simulink library "RIO_Lib"  (R2024b)
settings: Solver=VariableStepAuto  StartTime=0.0  StopTime=10.0  RelTol=1e-3
settings Model: Creator=pepev  LastModifiedBy=pepev

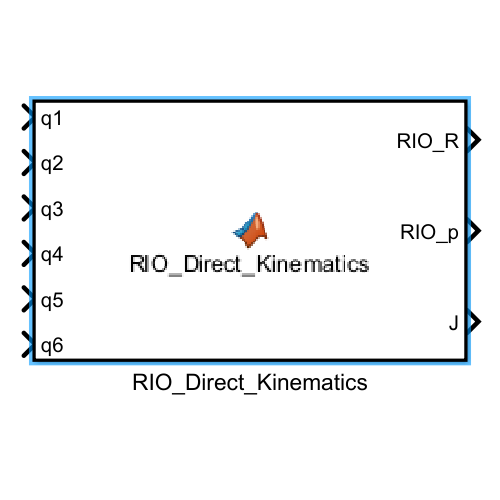
[thumbnail: Simulink's stored preview of the top-level diagram]
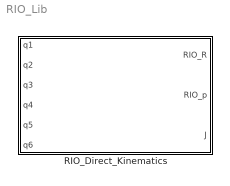
== system RIO_Lib ==
  RIO_Direct_Kinematics : MATLAB Function  TreatAsAtomicUnit=on

== matlab function RIO_Lib/RIO_Direct_Kinematics ==
  data: q1 input; RIO_R output; q2 input; q3 input; q4 input; q5 input; q6 input; RIO_p output; J output
function [RIO_R,RIO_p,J] = RIO_Direct_Kinematics(q1,q2,q3,q4,q5,q6)
%#codegen

%    This function was generated by the Symbolic Math Toolbox version 24.2.
%    20-May-2025 17:05:48

% q1 = complex(q1);  % if required to enforce complex operations
% q2 = complex(q2);  % if required to enforce complex operations
% q3 = complex(q3);  % if required to enforce complex operations
% q4 = complex(q4);  % if required to enforce complex operations
% q5 = complex(q5);  % if required to enforce complex operations
% q6 = complex(q6);  % if required to enforce complex operations
t2 = cos(q1);
t3 = cos(q2);
t4 = cos(q3);
t5 = cos(q4);
t6 = cos(q5);
t7 = cos(q6);
t8 = sin(q1);
t9 = sin(q2);
t10 = sin(q3);
t11 = sin(q4);
t12 = sin(q5);
t13 = sin(q6);
t14 = sqrt(2.0);
t15 = t9.*(3.0./1.0e+1);
t16 = t14+2.0;
t17 = (t9.*t11)./2.0;
t18 = -t14;
t19 = t2.*t3.*(3.0./1.0e+1);
t20 = t3.*t8.*(3.0./1.0e+1);
t21 = (t5.*t9)./1.0e+1;
t24 = (t2.*t4.*t5)./2.0;
t25 = (t2.*t3.*t11)./2.0;
t26 = (t4.*t5.*t8)./2.0;
t27 = (t3.*t5.*t10)./2.0;
t28 = (t3.*t8.*t11)./2.0;
t30 = (t2.*t3.*t5)./1.0e+1;
t31 = (t3.*t4.*t6)./1.0e+1;
t32 = (t3.*t5.*t8)./1.0e+1;
t33 = (t2.*t4.*t11)./1.0e+1;
t34 = (t2.*t6.*t10)./1.0e+1;
t36 = (t4.*t8.*t11)./1.0e+1;
t37 = (t3.*t10.*t11)./1.0e+1;
t38 = (t6.*t8.*t10)./1.0e+1;
t40 = (t2.*t5.*t9.*t10)./2.0;
t42 = (t5.*t8.*t9.*t10)./2.0;
t46 = (t2.*t4.*t6.*t9)./1.0e+1;
t48 = (t4.*t6.*t8.*t9)./1.0e+1;
t51 = (t2.*t9.*t10.*t11)./1.0e+1;
t54 = (t8.*t9.*t10.*t11)./1.0e+1;
t57 = t3.*t5.*t8.*t12.*(-1.0./1.0e+1);
t58 = t2.*t4.*t11.*t12.*(-1.0./1.0e+1);
t59 = t3.*t10.*t11.*t12.*(-1.0./1.0e+1);
t63 = t8.*t9.*t10.*t11.*t12.*(-1.0./1.0e+1);
t22 = -t20;
t23 = t18+2.0;
t29 = sqrt(t16);
t35 = -t28;
t39 = t12.*t21;
t41 = -t31;
t43 = -t32;
t44 = -t33;
t45 = -t37;
t47 = t12.*t30;
t50 = t12.*t33;
t52 = t12.*t36;
t56 = -t48;
t60 = -t54;
t61 = t12.*t51;
t55 = sqrt(t23);
mt1 = [t2.*t4.*t5.*t7-t3.*t7.*t8.*t11-t2.*t10.*t12.*t13-t3.*t5.*t6.*t8.*t13-t2.*t4.*t6.*t11.*t13+t5.*t7.*t8.*t9.*t10+t4.*t8.*t9.*t12.*t13-t6.*t8.*t9.*t10.*t11.*t13,t2.*t3.*t7.*t11+t4.*t5.*t7.*t8-t8.*t10.*t12.*t13+t2.*t3.*t5.*t6.*t13-t2.*t5.*t7.*t9.*t10-t2.*t4.*t9.*t12.*t13-t4.*t6.*t8.*t11.*t13+t2.*t6.*t9.*t10.*t11.*t13,t7.*t9.*t11+t3.*t5.*t7.*t10+t3.*t4.*t12.*t13+t5.*t6.*t9.*t13-t3.*t6.*t10.*t11.*t13];
mt2 = [t13.*t28.*t55-(t2.*t6.*t10.*t29)./2.0+(t4.*t6.*t8.*t9.*t29)./2.0+(t3.*t5.*t8.*t12.*t29)./2.0+(t2.*t4.*t11.*t12.*t29)./2.0+t8.*t10.*t12.*t17.*t29-(t2.*t4.*t5.*t13.*t55)./2.0-(t2.*t7.*t10.*t12.*t55)./2.0-(t3.*t5.*t6.*t7.*t8.*t55)./2.0-(t2.*t4.*t6.*t7.*t11.*t55)./2.0+(t4.*t7.*t8.*t9.*t12.*t55)./2.0-(t5.*t8.*t9.*t10.*t13.*t55)./2.0-(t6.*t7.*t8.*t9.*t10.*t11.*t55)./2.0];
mt3 = [t13.*t40.*t55-(t6.*t8.*t10.*t29)./2.0-(t2.*t4.*t6.*t9.*t29)./2.0-(t2.*t3.*t5.*t12.*t29)./2.0+(t4.*t8.*t11.*t12.*t29)./2.0-(t2.*t3.*t11.*t13.*t55)./2.0-(t4.*t5.*t8.*t13.*t55)./2.0-(t7.*t8.*t10.*t12.*t55)./2.0-(t2.*t9.*t10.*t11.*t12.*t29)./2.0+(t2.*t3.*t5.*t6.*t7.*t55)./2.0-(t2.*t4.*t7.*t9.*t12.*t55)./2.0-(t4.*t6.*t7.*t8.*t11.*t55)./2.0+t2.*t6.*t7.*t10.*t17.*t55,(t3.*t4.*t6.*t29)./2.0-(t5.*t9.*t12.*t29)./2.0-(t9.*t11.*t13.*t55)./2.0+(t3.*t10.*t11.*t12.*t29)./2.0+(t3.*t4.*t7.*t12.*t55)./2.0+(t5.*t6.*t7.*t9.*t55)./2.0-(t3.*t5.*t10.*t13.*t55)./2.0-(t3.*t6.*t7.*t10.*t11.*t55)./2.0];
mt4 = [t13.*t24.*t29+t13.*t29.*t42-(t2.*t6.*t10.*t55)./2.0+(t2.*t7.*t10.*t12.*t29)./2.0-(t3.*t8.*t11.*t13.*t29)./2.0+(t4.*t6.*t8.*t9.*t55)./2.0+(t3.*t5.*t8.*t12.*t55)./2.0+(t2.*t4.*t11.*t12.*t55)./2.0+t8.*t10.*t12.*t17.*t55+(t3.*t5.*t6.*t7.*t8.*t29)./2.0+(t2.*t4.*t6.*t7.*t11.*t29)./2.0-(t4.*t7.*t8.*t9.*t12.*t29)./2.0+t6.*t7.*t8.*t10.*t17.*t29];
mt5 = [t13.*t25.*t29+t13.*t26.*t29-(t6.*t8.*t10.*t55)./2.0+(t7.*t8.*t10.*t12.*t29)./2.0-(t2.*t4.*t6.*t9.*t55)./2.0-(t2.*t3.*t5.*t12.*t55)./2.0+(t4.*t8.*t11.*t12.*t55)./2.0-(t2.*t3.*t5.*t6.*t7.*t29)./2.0+(t2.*t4.*t7.*t9.*t12.*t29)./2.0+(t4.*t6.*t7.*t8.*t11.*t29)./2.0-(t2.*t5.*t9.*t10.*t13.*t29)./2.0-(t2.*t9.*t10.*t11.*t12.*t55)./2.0-(t2.*t6.*t7.*t9.*t10.*t11.*t29)./2.0,t13.*t17.*t29+t13.*t27.*t29+(t3.*t4.*t6.*t55)./2.0-(t5.*t9.*t12.*t55)./2.0-(t3.*t4.*t7.*t12.*t29)./2.0-(t5.*t6.*t7.*t9.*t29)./2.0+(t3.*t10.*t11.*t12.*t55)./2.0+(t3.*t6.*t7.*t10.*t11.*t29)./2.0];
RIO_R = reshape([mt1,mt2,mt3,mt4,mt5],3,3);
if nargout > 1
    t64 = t9.*t11.*t13.*t29.*(2.3e+1./4.0e+2);
    t65 = t2.*t4.*t5.*t13.*t29.*(2.3e+1./4.0e+2);
    t66 = t3.*t4.*t7.*t12.*t29.*(2.3e+1./4.0e+2);
    t67 = t5.*t6.*t7.*t9.*t29.*(2.3e+1./4.0e+2);
    t68 = t2.*t3.*t11.*t13.*t29.*(2.3e+1./4.0e+2);
    t69 = t4.*t5.*t8.*t13.*t29.*(2.3e+1./4.0e+2);
    t70 = t2.*t7.*t10.*t12.*t29.*(2.3e+1./4.0e+2);
    t71 = t3.*t5.*t10.*t13.*t29.*(2.3e+1./4.0e+2);
    t72 = t3.*t8.*t11.*t13.*t29.*(2.3e+1./4.0e+2);
    t73 = t7.*t8.*t10.*t12.*t29.*(2.3e+1./4.0e+2);
    t83 = t2.*t3.*t5.*t6.*t7.*t29.*(2.3e+1./4.0e+2);
    t84 = t3.*t5.*t6.*t7.*t8.*t29.*(2.3e+1./4.0e+2);
    t85 = t2.*t4.*t6.*t7.*t11.*t29.*(2.3e+1./4.0e+2);
    t86 = t2.*t4.*t7.*t9.*t12.*t29.*(2.3e+1./4.0e+2);
    t87 = t4.*t6.*t7.*t8.*t11.*t29.*(2.3e+1./4.0e+2);
    t88 = t3.*t6.*t7.*t10.*t11.*t29.*(2.3e+1./4.0e+2);
    t89 = t2.*t5.*t9.*t10.*t13.*t29.*(2.3e+1./4.0e+2);
    t90 = t4.*t7.*t8.*t9.*t12.*t29.*(2.3e+1./4.0e+2);
    t91 = t5.*t8.*t9.*t10.*t13.*t29.*(2.3e+1./4.0e+2);
    t100 = t2.*t6.*t7.*t9.*t10.*t11.*t29.*(2.3e+1./4.0e+2);
    t101 = t6.*t7.*t8.*t9.*t10.*t11.*t29.*(2.3e+1./4.0e+2);
    t74 = t3.*t4.*t6.*t55.*(2.3e+1./4.0e+2);
    t75 = t2.*t6.*t10.*t55.*(2.3e+1./4.0e+2);
    t76 = t6.*t8.*t10.*t55.*(2.3e+1./4.0e+2);
    t77 = t5.*t9.*t12.*t55.*(2.3e+1./4.0e+2);
    t78 = -t66;
    t79 = -t67;
    t80 = -t72;
    t92 = t2.*t4.*t6.*t9.*t55.*(2.3e+1./4.0e+2);
    t93 = t2.*t3.*t5.*t12.*t55.*(2.3e+1./4.0e+2);
    t94 = t4.*t6.*t8.*t9.*t55.*(2.3e+1./4.0e+2);
    t95 = t3.*t5.*t8.*t12.*t55.*(2.3e+1./4.0e+2);
    t96 = t2.*t4.*t11.*t12.*t55.*(2.3e+1./4.0e+2);
    t97 = t4.*t8.*t11.*t12.*t55.*(2.3e+1./4.0e+2);
    t98 = t3.*t10.*t11.*t12.*t55.*(2.3e+1./4.0e+2);
    t99 = -t90;
    t102 = t2.*t9.*t10.*t11.*t12.*t55.*(2.3e+1./4.0e+2);
    t103 = t8.*t9.*t10.*t11.*t12.*t55.*(2.3e+1./4.0e+2);
    t81 = -t75;
    t82 = -t77;
    t104 = t15+t17+t21+t27+t39+t41+t45+t59+t64+t71+t74+t78+t79+t82+t88+t98;
    t105 = t22+t24+t34+t35+t42+t43+t44+t56+t57+t58+t60+t63+t65+t70+t80+t81+t84+t85+t91+t94+t95+t96+t99+t101+t103;
    RIO_p = [t105;t19+t25+t26+t30-t36+t38-t40+t46+t47+t51+t61+t68+t69+t73-t76-t83+t86+t87-t89-t92-t93+t97-t100-t102-(t4.*t8.*t11.*t12)./1.0e+1;t104];
end
if nargout > 2
    mt6 = [-t19-t25-t26-t30+t36-t38+t40-t46-t51+t52-t68-t69-t73+t76+t83-t86-t87+t89+t92+t93-t97+t100+t102-(t2.*t3.*t5.*t12)./1.0e+1-(t2.*t9.*t10.*t11.*t12)./1.0e+1,t105,0.0,0.0,0.0,1.0,t8.*t104,-t2.*t104];
    mt7 = [t3.*(3.0./1.0e+1)+(t3.*t5)./1.0e+1+(t3.*t11)./2.0+(t4.*t6.*t9)./1.0e+1+(t3.*t5.*t12)./1.0e+1-(t5.*t9.*t10)./2.0+(t9.*t10.*t11)./1.0e+1+(t9.*t10.*t11.*t12)./1.0e+1+t3.*t11.*t13.*t29.*(2.3e+1./4.0e+2)-t4.*t6.*t9.*t55.*(2.3e+1./4.0e+2)-t3.*t5.*t12.*t55.*(2.3e+1./4.0e+2)-t3.*t5.*t6.*t7.*t29.*(2.3e+1./4.0e+2)+t4.*t7.*t9.*t12.*t29.*(2.3e+1./4.0e+2)-t5.*t9.*t10.*t13.*t29.*(2.3e+1./4.0e+2)-t9.*t10.*t11.*t12.*t55.*(2.3e+1./4.0e+2)-t6.*t7.*t9.*t10.*t11.*t29.*(2.3e+1./4.0e+2),t2,t8,0.0];
    mt8 = [t9.*t26+t9.*t38+t9.*t69+t9.*t73+t9.*t87+t9.*t97+(t2.*t4.*t6)./1.0e+1-(t2.*t5.*t10)./2.0+(t2.*t10.*t11)./1.0e+1-(t4.*t8.*t9.*t11)./1.0e+1+(t2.*t10.*t11.*t12)./1.0e+1-t2.*t4.*t6.*t55.*(2.3e+1./4.0e+2)-(t4.*t8.*t9.*t11.*t12)./1.0e+1+t2.*t4.*t7.*t12.*t29.*(2.3e+1./4.0e+2)-t2.*t5.*t10.*t13.*t29.*(2.3e+1./4.0e+2)-t6.*t8.*t9.*t10.*t55.*(2.3e+1./4.0e+2)-t2.*t10.*t11.*t12.*t55.*(2.3e+1./4.0e+2)-t2.*t6.*t7.*t10.*t11.*t29.*(2.3e+1./4.0e+2)];
    mt9 = [t9.*t33+t9.*t50+t9.*t75+(t4.*t6.*t8)./1.0e+1-(t5.*t8.*t10)./2.0+(t8.*t10.*t11)./1.0e+1-(t2.*t4.*t5.*t9)./2.0-(t2.*t6.*t9.*t10)./1.0e+1+(t8.*t10.*t11.*t12)./1.0e+1-t4.*t6.*t8.*t55.*(2.3e+1./4.0e+2)+t4.*t7.*t8.*t12.*t29.*(2.3e+1./4.0e+2)-t5.*t8.*t10.*t13.*t29.*(2.3e+1./4.0e+2)-t8.*t10.*t11.*t12.*t55.*(2.3e+1./4.0e+2)-t2.*t4.*t5.*t9.*t13.*t29.*(2.3e+1./4.0e+2)-t2.*t7.*t9.*t10.*t12.*t29.*(2.3e+1./4.0e+2)-t6.*t7.*t8.*t10.*t11.*t29.*(2.3e+1./4.0e+2)-t2.*t4.*t9.*t11.*t12.*t55.*(2.3e+1./4.0e+2)-t2.*t4.*t6.*t7.*t9.*t11.*t29.*(2.3e+1./4.0e+2)];
    mt10 = [(t3.*(t4.*t5.*2.0e+2-t4.*t11.*4.0e+1+t6.*t10.*4.0e+1-t4.*t11.*t12.*4.0e+1-t6.*t10.*t55.*2.3e+1+t4.*t5.*t13.*t29.*2.3e+1+t7.*t10.*t12.*t29.*2.3e+1+t4.*t11.*t12.*t55.*2.3e+1+t4.*t6.*t7.*t11.*t29.*2.3e+1))./4.0e+2,t3.*t8,-t2.*t3,-t9];
    mt11 = [t2.*t4.*t5.*(-1.0./1.0e+1)-(t3.*t5.*t8)./2.0-(t2.*t4.*t11)./2.0+(t3.*t8.*t11)./1.0e+1+t8.*t10.*t67+t8.*t10.*t77-(t2.*t4.*t5.*t12)./1.0e+1-(t5.*t8.*t9.*t10)./1.0e+1+(t3.*t8.*t11.*t12)./1.0e+1-(t8.*t9.*t10.*t11)./2.0-(t5.*t8.*t9.*t10.*t12)./1.0e+1-t3.*t5.*t8.*t13.*t29.*(2.3e+1./4.0e+2)-t2.*t4.*t11.*t13.*t29.*(2.3e+1./4.0e+2)+t2.*t4.*t5.*t12.*t55.*(2.3e+1./4.0e+2)-t3.*t8.*t11.*t12.*t55.*(2.3e+1./4.0e+2)+t2.*t4.*t5.*t6.*t7.*t29.*(2.3e+1./4.0e+2)-t3.*t6.*t7.*t8.*t11.*t29.*(2.3e+1./4.0e+2)-t8.*t9.*t10.*t11.*t13.*t29.*(2.3e+1./4.0e+2)];
    mt12 = [(t2.*t3.*t5)./2.0-(t2.*t3.*t11)./1.0e+1-(t4.*t5.*t8)./1.0e+1-(t4.*t8.*t11)./2.0+t2.*t10.*t17+t2.*t10.*t21+t2.*t10.*t39+t2.*t10.*t64-(t2.*t3.*t11.*t12)./1.0e+1-(t4.*t5.*t8.*t12)./1.0e+1+t2.*t3.*t5.*t13.*t29.*(2.3e+1./4.0e+2)-t4.*t8.*t11.*t13.*t29.*(2.3e+1./4.0e+2)+t2.*t3.*t11.*t12.*t55.*(2.3e+1./4.0e+2)+t4.*t5.*t8.*t12.*t55.*(2.3e+1./4.0e+2)+t2.*t3.*t6.*t7.*t11.*t29.*(2.3e+1./4.0e+2)+t4.*t5.*t6.*t7.*t8.*t29.*(2.3e+1./4.0e+2)-t2.*t5.*t9.*t10.*t12.*t55.*(2.3e+1./4.0e+2)-t2.*t5.*t6.*t7.*t9.*t10.*t29.*(2.3e+1./4.0e+2)];
    mt13 = [(t5.*t9)./2.0-(t9.*t11)./1.0e+1-(t3.*t5.*t10)./1.0e+1-(t3.*t10.*t11)./2.0-(t9.*t11.*t12)./1.0e+1-(t3.*t5.*t10.*t12)./1.0e+1+t5.*t9.*t13.*t29.*(2.3e+1./4.0e+2)+t9.*t11.*t12.*t55.*(2.3e+1./4.0e+2)+t6.*t7.*t9.*t11.*t29.*(2.3e+1./4.0e+2)-t3.*t10.*t11.*t13.*t29.*(2.3e+1./4.0e+2)+t3.*t5.*t10.*t12.*t55.*(2.3e+1./4.0e+2)+t3.*t5.*t6.*t7.*t10.*t29.*(2.3e+1./4.0e+2),-t2.*t10+t4.*t8.*t9,-t8.*t10-t2.*t4.*t9,t3.*t4];
    mt14 = [t2.*t10.*t12.*(-1.0./1.0e+1)+t9.*t11.*t76-(t3.*t5.*t6.*t8)./1.0e+1-(t2.*t4.*t6.*t11)./1.0e+1+(t4.*t8.*t9.*t12)./1.0e+1+t2.*t10.*t12.*t55.*(2.3e+1./4.0e+2)-(t6.*t8.*t9.*t10.*t11)./1.0e+1+t2.*t6.*t7.*t10.*t29.*(2.3e+1./4.0e+2)+t3.*t5.*t6.*t8.*t55.*(2.3e+1./4.0e+2)+t2.*t4.*t6.*t11.*t55.*(2.3e+1./4.0e+2)-t4.*t8.*t9.*t12.*t55.*(2.3e+1./4.0e+2)-t4.*t6.*t7.*t8.*t9.*t29.*(2.3e+1./4.0e+2)-t3.*t5.*t7.*t8.*t12.*t29.*(2.3e+1./4.0e+2)-t2.*t4.*t7.*t11.*t12.*t29.*(2.3e+1./4.0e+2)-t7.*t8.*t9.*t10.*t11.*t12.*t29.*(2.3e+1./4.0e+2)];
    mt15 = [t6.*t30-(t8.*t10.*t12)./1.0e+1+t9.*t11.*t34+t9.*t11.*t70-(t2.*t4.*t9.*t12)./1.0e+1-(t4.*t6.*t8.*t11)./1.0e+1+t8.*t10.*t12.*t55.*(2.3e+1./4.0e+2)+t6.*t7.*t8.*t10.*t29.*(2.3e+1./4.0e+2)-t2.*t3.*t5.*t6.*t55.*(2.3e+1./4.0e+2)+t2.*t4.*t9.*t12.*t55.*(2.3e+1./4.0e+2)+t4.*t6.*t8.*t11.*t55.*(2.3e+1./4.0e+2)+t2.*t4.*t6.*t7.*t9.*t29.*(2.3e+1./4.0e+2)+t2.*t3.*t5.*t7.*t12.*t29.*(2.3e+1./4.0e+2)-t4.*t7.*t8.*t11.*t12.*t29.*(2.3e+1./4.0e+2)-t2.*t6.*t9.*t10.*t11.*t55.*(2.3e+1./4.0e+2)];
    mt16 = [t6.*t21+(t3.*t4.*t12)./1.0e+1-(t3.*t6.*t10.*t11)./1.0e+1-t3.*t4.*t12.*t55.*(2.3e+1./4.0e+2)-t5.*t6.*t9.*t55.*(2.3e+1./4.0e+2)-t3.*t4.*t6.*t7.*t29.*(2.3e+1./4.0e+2)+t5.*t7.*t9.*t12.*t29.*(2.3e+1./4.0e+2)+t3.*t6.*t10.*t11.*t55.*(2.3e+1./4.0e+2)-t3.*t7.*t10.*t11.*t12.*t29.*(2.3e+1./4.0e+2),t2.*t4.*t5-t3.*t8.*t11+t5.*t8.*t9.*t10,t2.*t3.*t11+t4.*t5.*t8-t2.*t5.*t9.*t10,t9.*t11+t3.*t5.*t10];
    mt17 = [t2.*t4.*t5.*t7.*t29.*(2.3e+1./4.0e+2)-t3.*t7.*t8.*t11.*t29.*(2.3e+1./4.0e+2)-t2.*t10.*t12.*t13.*t29.*(2.3e+1./4.0e+2)-t3.*t5.*t6.*t8.*t13.*t29.*(2.3e+1./4.0e+2)-t2.*t4.*t6.*t11.*t13.*t29.*(2.3e+1./4.0e+2)+t5.*t7.*t8.*t9.*t10.*t29.*(2.3e+1./4.0e+2)+t4.*t8.*t9.*t12.*t13.*t29.*(2.3e+1./4.0e+2)-t6.*t8.*t9.*t10.*t11.*t13.*t29.*(2.3e+1./4.0e+2)];
    mt18 = [t2.*t6.*t10.*t64+t2.*t3.*t7.*t11.*t29.*(2.3e+1./4.0e+2)+t4.*t5.*t7.*t8.*t29.*(2.3e+1./4.0e+2)-t8.*t10.*t12.*t13.*t29.*(2.3e+1./4.0e+2)+t2.*t3.*t5.*t6.*t13.*t29.*(2.3e+1./4.0e+2)-t2.*t5.*t7.*t9.*t10.*t29.*(2.3e+1./4.0e+2)-t2.*t4.*t9.*t12.*t13.*t29.*(2.3e+1./4.0e+2)-t4.*t6.*t8.*t11.*t13.*t29.*(2.3e+1./4.0e+2),t7.*t9.*t11.*t29.*(2.3e+1./4.0e+2)+t3.*t5.*t7.*t10.*t29.*(2.3e+1./4.0e+2)+t3.*t4.*t12.*t13.*t29.*(2.3e+1./4.0e+2)+t5.*t6.*t9.*t13.*t29.*(2.3e+1./4.0e+2)-t3.*t6.*t10.*t11.*t13.*t29.*(2.3e+1./4.0e+2),-t2.*t6.*t10+t4.*t6.*t8.*t9+t3.*t5.*t8.*t12+t2.*t4.*t11.*t12+t8.*t9.*t10.*t11.*t12];
    mt19 = [-t6.*t8.*t10-t2.*t4.*t6.*t9-t2.*t3.*t5.*t12+t4.*t8.*t11.*t12-t2.*t9.*t10.*t11.*t12,t3.*t4.*t6-t5.*t9.*t12+t3.*t10.*t11.*t12];
    J = reshape([mt6,mt7,mt8,mt9,mt10,mt11,mt12,mt13,mt14,mt15,mt16,mt17,mt18,mt19],6,6);
end
end
